simulink model "tarmodel"  (R2015a)
settings: Solver=ode3  SolverMode=SingleTasking  StartTime=0.0  StopTime=10.0  RelTol=1e-3
Description:
  | ###CmwHarnessModel###
settings Model: CovMetricSettings=dwe  CovHtmlReporting=off  covSaveCumulativeToWorkspaceVar=off  CovSaveSingleToWorkspaceVar=off  CovExternalEMLEnable=on  Creator=chin.j  LastModifiedBy=user2.gaio
settings DataIOCC: LimitDataPoints=off  SaveFormat=Dataset  SaveOutput=off  SaveTime=off
settings DebuggingCC: StrictBusMsg=ErrorOnBusTreatedAsVector  SFUnexpectedBacktrackingDiag=error  SFNoUnconditionalDefaultTransitionDiag=error
settings HardwareCC: ProdBitPerPointer=64  ProdLargestAtomicFloat=Float  ProdIntDivRoundTo=Zero  ProdEndianess=LittleEndian  ProdHWDeviceType=Specified
settings ModelReferenceCC: PropagateSignalLabelsOutOfModel=on
settings SFSimCC: SimUseLocalCustomCode=on
settings RTWCC: RTWUseLocalCustomCode=on
settings GRTTargetCC: TargetLangStandard=C99 (ISO)  GeneratePreprocessorConditionals=Use local settings

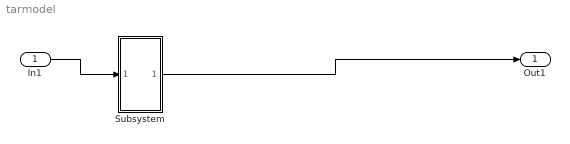
== system tarmodel ==
  In1 : Inport  OutDataTypeStr=double  PortDimensions=1  Interpolate=off
  Subsystem : Subsystem
  Out1 : Outport  OutDataTypeStr=double
  wires:
  In1/1 -> Subsystem/1(In1)
  Subsystem/1(Out1) -> Out1/1

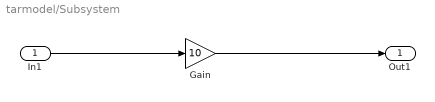
== system tarmodel/Subsystem ==
  In1 : Inport
  Gain : Gain  Gain=10
  Out1 : Outport
  wires:
  In1/1 -> Gain/1
  Gain/1 -> Out1/1
